simulink library "groundStationPrescribed001_cl"  (R2020a)
settings: Solver=VariableStepAuto  StartTime=0.0  StopTime=10.0  RelTol=1e-3
undefined symbols (not defined in the file): gndStn
libraries: simulink x1, eulAng2RotMat_ul x1, firstOrdTrnsThm_ul x1
settings Model: Creator=M.Cobb  LastModifiedBy=andre
settings DataIOCC: ReturnWorkspaceOutputs=off
settings DebuggingCC: ArithmeticOperatorsInVariantConditions=warning
settings SFSimCC: CustomCodeUndefinedFunction=UseInterfaceOnly

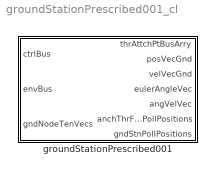
== system groundStationPrescribed001_cl ==
  groundStationPrescribed001 : Subsystem  mask{gs=0}
      mask prompts: gs "Ground station object"

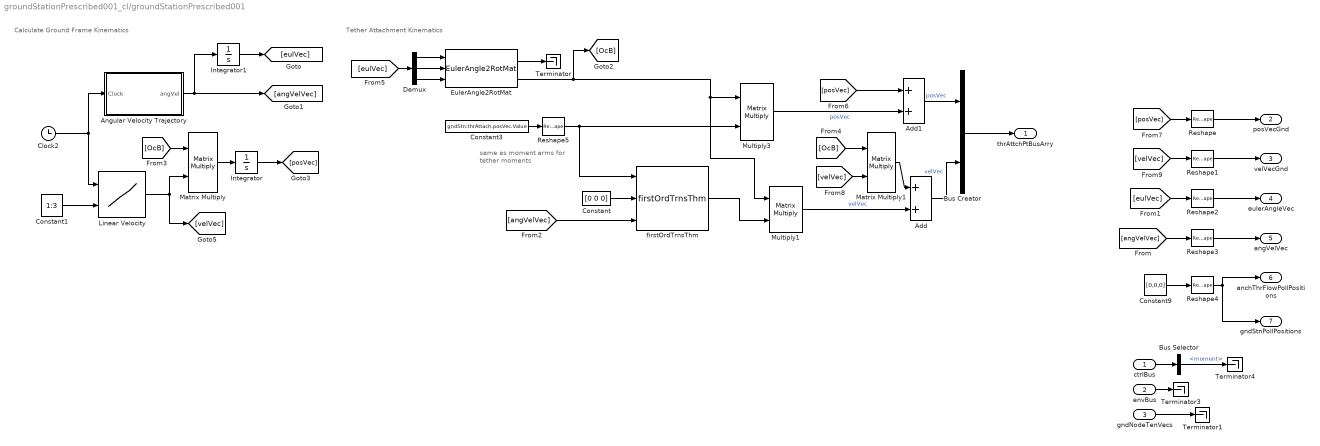
== system groundStationPrescribed001_cl/groundStationPrescribed001 ==
  note: Tether Attachment Kinematics
  note: Calculate Ground Frame Kinematics
  note: same as moment arms
      | for tether moments
  ctrlBus : Inport  OutDataTypeStr=Bus: gndStnCtrlBus
  envBus : Inport  Port=2  OutDataTypeStr=Bus: envBus
  gndNodeTenVecs : Inport  Port=3
  Add : Sum
  Add1 : Sum
  Angular Velocity Trajectory : Subsystem
  Bus Creator : BusCreator  Inputs=2  OutDataTypeStr=Bus: thrAttachPtKinematicsBus  NonVirtualBus=on
  Bus Selector : BusSelector  OutputSignals=moment
  Clock2 : Clock
  Constant : Constant  Value=[0 0 0]
  Constant1 : Constant  Value=1:3
  Constant3 : Constant  Value=gndStn.thrAttach.posVec.Value
  Constant9 : Constant  Value=[0,0,0]
  Demux : Demux  Outputs=3
  EulerAngle2RotMat : eulAng2RotMat_ul/EulerAngle2RotMat  SystemSampleTime=-1  Latency=0  AutoFrameSizeCalculation=off
  Integrator : Integrator  InitialCondition=gndStn.initPosVecGnd.Value
  Integrator1 : Integrator  InitialCondition=gndStn.initEulAng.Value
  Linear Velocity : Lookup_n-D  BreakpointsForDimension1=gndStn.velVecTrajectory.Value.Time  BreakpointsForDimension2=[1:3]  BreakpointsForDimension3=[5, 7]  Table=gndStn.velVecTrajectory.Value.Data  InternalRulePriority=Speed  RndMeth=Simplest
  Matrix Multiply : Product  Multiplication=Matrix(*)
  Matrix Multiply1 : Product  Multiplication=Matrix(*)
  Multiply1 : Product  Multiplication=Matrix(*)
  Multiply3 : Product  Multiplication=Matrix(*)
  Reshape{,1..5} (6 alike) : Reshape  OutputDimensionality=Column vector (2-D)
  Terminator{,1,3..4} (4 alike) : Terminator
  firstOrdTrnsThm : firstOrdTrnsThm_ul/firstOrdTrnsThm  SystemSampleTime=-1  Latency=0  AutoFrameSizeCalculation=off
  thrAttchPtBusArry : Outport  VectorParamsAs1DForOutWhenUnconnected=off
  posVecGnd : Outport  Port=2  VectorParamsAs1DForOutWhenUnconnected=off
  velVecGnd : Outport  Port=3  VectorParamsAs1DForOutWhenUnconnected=off
  eulerAngleVec : Outport  Port=4  VectorParamsAs1DForOutWhenUnconnected=off
  angVelVec : Outport  Port=5  VectorParamsAs1DForOutWhenUnconnected=off
  anchThrFlowPollPositions : Outport  Port=6  VectorParamsAs1DForOutWhenUnconnected=off
  gndStnPollPositions : Outport  Port=7  VectorParamsAs1DForOutWhenUnconnected=off
  wires:
  ctrlBus/1 -> Bus Selector/1
  envBus/1 -> Terminator3/1
  gndNodeTenVecs/1 -> Terminator1/1
  Reshape/1 -> posVecGnd/1
  Reshape1/1 -> velVecGnd/1
  Reshape2/1 -> eulerAngleVec/1
  Reshape3/1 -> angVelVec/1
  [angVelVec] -> Reshape3/1
  Bus Selector/1 -> Terminator4/1  "<moment>"
  Reshape4/1 -> anchThrFlowPollPositions/1, gndStnPollPositions/1
  Constant9/1 -> Reshape4/1
  [posVec] -> Reshape/1
  [velVec] -> Reshape1/1
  Linear Velocity/1 -> Matrix Multiply/2, [velVec]
  Constant1/1 -> Linear Velocity/2
  [eulVec] -> Reshape2/1
  EulerAngle2RotMat/1 -> Terminator/1
  Integrator1/1 -> [eulVec]
  Demux/3 -> EulerAngle2RotMat/3
  Demux/2 -> EulerAngle2RotMat/2
  Demux/1 -> EulerAngle2RotMat/1
  Add1/1 -> Bus Creator/1  "posVec"
  Constant/1 -> firstOrdTrnsThm/2
  Constant3/1 -> Reshape5/1
  firstOrdTrnsThm/1 -> Multiply1/2
  Reshape5/1 -> firstOrdTrnsThm/1, Multiply3/2
  Add/1 -> Bus Creator/2  "velVec"
  EulerAngle2RotMat/2 -> [OcB], Multiply1/1, Multiply3/1
  [velVec] -> Matrix Multiply1/2
  [posVec] -> Add1/1
  Multiply3/1 -> Add1/2  "posVec"
  Multiply1/1 -> Add/2  "velVec"
  Bus Creator/1 -> thrAttchPtBusArry/1
  [angVelVec] -> firstOrdTrnsThm/3
  [OcB] -> Matrix Multiply/1
  Matrix Multiply/1 -> Integrator/1
  Integrator/1 -> [posVec]
  Angular Velocity Trajectory/1(angVel) -> Integrator1/1, [angVelVec]
  Clock2/1 -> Angular Velocity Trajectory/1(Clock), Linear Velocity/1
  [OcB] -> Matrix Multiply1/1
  [eulVec] -> Demux/1
  Matrix Multiply1/1 -> Add/1

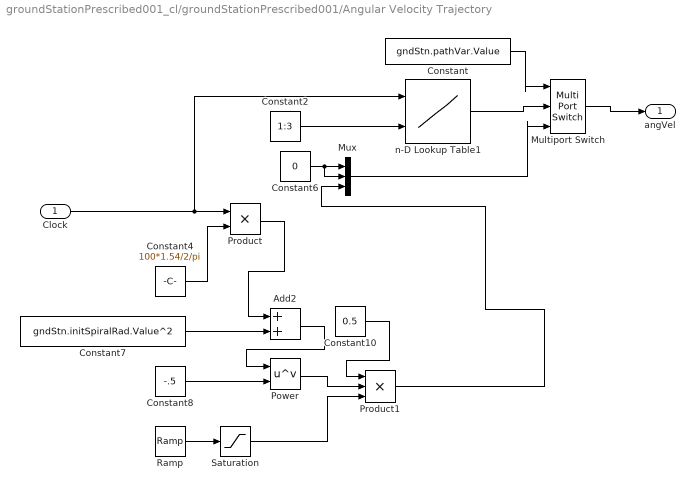
== system groundStationPrescribed001_cl/groundStationPrescribed001/Angular Velocity Trajectory ==
  Clock : Inport
  Add2 : Sum
  Constant : Constant  Value=gndStn.pathVar.Value
  Constant10 : Constant  Value=0.5
  Constant2 : Constant  Value=1:3
  Constant4 : Constant  Value=100*1.54/2/pi
  Constant6 : Constant  Value=0
  Constant7 : Constant  Value=gndStn.initSpiralRad.Value^2
  Constant8 : Constant  Value=-.5
  Multiport Switch : MultiPortSwitch  Inputs=2
  Mux : Mux  Inputs=3
  Power : Math  Operator=pow  SaturateOnIntegerOverflow=on
  Product : Product
  Product1 : Product  Inputs=3
  Ramp : simulink/Sources/Ramp  slope=1/30  start=0  InitialOutput=0
  Saturation : Saturate  UpperLimit=1
  n-D Lookup Table1 : Lookup_n-D  BreakpointsForDimension1=gndStn.angVelTrajectory.Value.Time  BreakpointsForDimension2=[1:3]  BreakpointsForDimension3=[5, 7]  Table=gndStn.angVelTrajectory.Value.Data  InternalRulePriority=Speed  RndMeth=Simplest  InputSameDT=on
  angVel : Outport
  wires:
  Constant8/1 -> Power/2
  Constant4/1 -> Product/2
  Product1/1 -> Mux/3
  Product/1 -> Add2/1
  Saturation/1 -> Product1/3
  Constant7/1 -> Add2/2
  Add2/1 -> Power/1
  Constant2/1 -> n-D Lookup Table1/2
  Constant6/1 -> Mux/2, Mux/1
  Power/1 -> Product1/2
  Ramp/1 -> Saturation/1
  Clock/1 -> n-D Lookup Table1/1, Product/1
  Constant10/1 -> Product1/1
  n-D Lookup Table1/1 -> Multiport Switch/2
  Mux/1 -> Multiport Switch/3
  Multiport Switch/1 -> angVel/1
  Constant/1 -> Multiport Switch/1
